simulink model "ROS2ValetVehicleExample"  (R2022b)
settings: Solver=FixedStepAuto  StartTime=0.0  StopTime=inf  FixedStep=0.05  MaxStep=1e-2  MinStep=1e-3  RelTol=5e-3
StopFcn:
  | exampleHelperROSValetModelCallbacks('stopfcn');
model workspace (MAT data in the model file):
  SL_ROS_VariableLengthArrays_MaxSizes.CommonInfo.ArrayTruncateAction = 'EmitWarning'
  SL_ROS_VariableLengthArrays_MaxSizes.MsgTypeMap = containers.Map
  SL_ROS_VariableLengthArrays_MaxSizes.MsgTypeMap.serialization.keys = {'std_msgs/Float64MultiArray'}
  SL_ROS_VariableLengthArrays_MaxSizes.MsgTypeMap.serialization.values{1}.PropertyName = 'data'
  SL_ROS_VariableLengthArrays_MaxSizes.MsgTypeMap.serialization.values{1}.DataType = 'double'
  SL_ROS_VariableLengthArrays_MaxSizes.MsgTypeMap.serialization.values{1}.MaxLength = 1500
  SL_ROS_VariableLengthArrays_MaxSizes.MsgTypeMap.serialization.uniformity = 0
  SL_ROS_VariableLengthArrays_MaxSizes.MsgTypeMap.serialization.keyType = 'char'
  SL_ROS_VariableLengthArrays_MaxSizes.MsgTypeMap.serialization.valueType = 'any'
values from neighbouring files (symbols this model uses):
  costmapStruct = rmfield(costmapStruct, 'CollisionChecker')    [exampleHelperROSValetSLCreateUtilityStruct.m]
  vehicleDimsStruct = exampleHelperROSValetMatchStructFields(vehicleDimsStruct, obj.CollisionChecker.VehicleDimensions)    [exampleHelperROSValetSLCreateUtilityStruct.m]
undefined symbols (not defined in the file or in its folder): startPose, theta, x, y
libraries: ros2lib x15, simulink x2, simulink_extras x2, helperVarsizeLib x1, autolibshared x1
CloseFcn:
  | exampleHelperROSValetModelCallbacks('closefcn');
settings Model: Creator=The MathWorks, Inc.  LastModifiedBy=The MathWorks, Inc.
settings SolverCC: ZeroCrossAlgorithm=Adaptive  AlgebraicLoopSolver=TrustRegion
settings OptimizationCC: EnhancedBackFolding=on  PassReuseOutputArgsThreshold=0  ZeroExternalMemoryAtStartup=off  ZeroInternalMemoryAtStartup=off  MaxStackSize=64  OptimizeBlockOrder=speed  DifferentSizesBufferReuse=on  OptimizationCustomize=off
settings DebuggingCC: ParameterTunabilityLossMsg=error  UnconnectedInputMsg=warning  UnconnectedOutputMsg=warning  UnconnectedLineMsg=warning  SFMachineParentedDataDiag=warning
settings HardwareCC: UseEmbeddedCoderFeatures=off
settings ModelReferenceCC: EnableRefExpFcnMdlSchedulingChecks=on
settings SFSimCC: MATLABDynamicMemAlloc=off  SimTargetLang=C++
settings RTWCC: Description=Embedded Coder  SystemTargetFile=ert.tlc  HardwareBoard=Robot Operating System 2 (ROS 2)  TLCOptions=-aInlineSetEventsForThisBaseRateFcn=TLC_FALSE -aSuppressMultiTaskScheduler=TLC_FALSE -aRateBasedStepFcn=1  TemplateMakefile=ert_default_tmf  GenerateReport=on  Toolchain=Colcon Tools  LaunchReport=on  TargetLang=C++
settings CodeAppCC: ForceParamTrailComments=on  OperatorAnnotations=on
settings ERTTargetCC: ERTCustomFileBanners=off  CodeInterfacePackaging=C++ class  SupportContinuousTime=on  SupportNonInlinedSFcns=on  RemoveResetFunc=off  ModelStepFunctionPrototypeControlCompliant=off  RootIOFormat=Structure reference

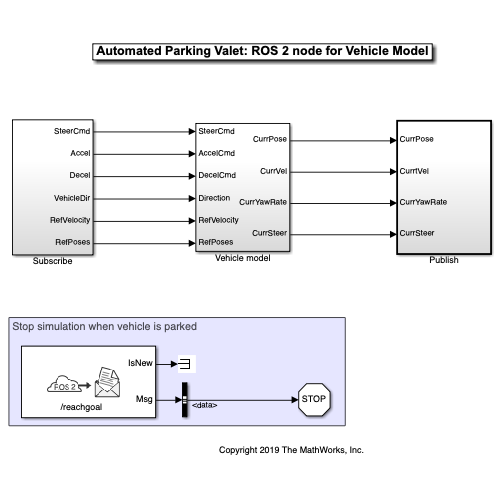
[thumbnail: Simulink's stored preview of the top-level diagram]
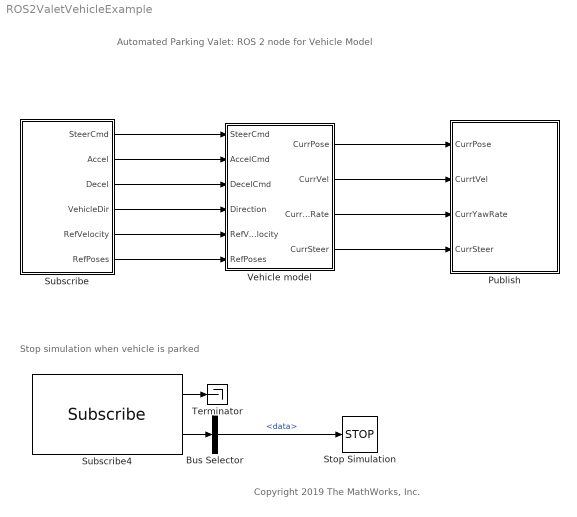
== system ROS2ValetVehicleExample ==
  note: Automated Parking Valet: ROS 2 node for Vehicle Model
  note: Copyright 2019 The MathWorks, Inc.
  note: Stop simulation when vehicle is parked
  Bus Selector : BusSelector  OutputSignals=data
  Publish : Subsystem  TreatAsAtomicUnit=on
  Stop Simulation : Stop
  Subscribe : Subsystem  SystemSampleTime=0.01
  Subscribe4 : ros2lib/Subscribe  topicSource=Specify your own  topic=/reachgoal  messageType=std_msgs/Bool  sampleTime=-1  QOSHistory=Keep last  QOSDepth=1  QOSReliability=Reliable  QOSDurability=Volatile
  Terminator : Terminator
  Vehicle model : Subsystem
  wires:
  Subscribe/1(SteerCmd) -> Vehicle model/1(SteerCmd)
  Subscribe/2(Accel) -> Vehicle model/2(AccelCmd)
  Subscribe/3(Decel) -> Vehicle model/3(DecelCmd)
  Subscribe/4(VehicleDir) -> Vehicle model/4(Direction)
  Subscribe/6(RefPoses) -> Vehicle model/6(RefPoses)
  Subscribe/5(RefVelocity) -> Vehicle model/5(RefVelocity)
  Vehicle model/1(CurrPose) -> Publish/1(CurrPose)
  Vehicle model/2(CurrVel) -> Publish/2(CurrtVel)
  Vehicle model/3(CurrYawRate) -> Publish/3(CurrYawRate)
  Vehicle model/4(CurrSteer) -> Publish/4(CurrSteer)
  Bus Selector/1 -> Stop Simulation/1  "<data>"
  Subscribe4/1 -> Terminator/1
  Subscribe4/2 -> Bus Selector/1

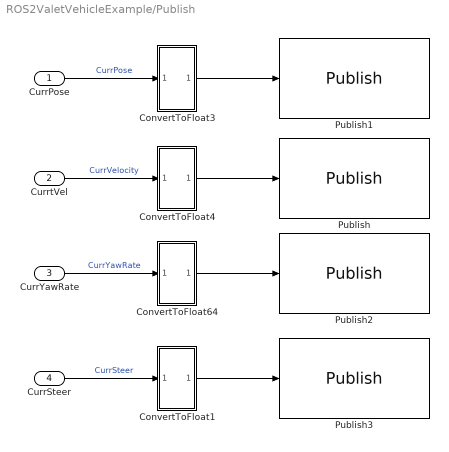
== system ROS2ValetVehicleExample/Publish ==
  CurrPose : Inport
  CurrtVel : Inport  Port=2
  CurrYawRate : Inport  Port=3
  CurrSteer : Inport  Port=4
  ConvertToFloat1 : Subsystem
  ConvertToFloat3 : Subsystem
  ConvertToFloat4 : Subsystem
  ConvertToFloat64 : Subsystem
  Publish : ros2lib/Publish  topicSource=Specify your own  topic=/currentvel  messageType=std_msgs/Float64  QOSHistory=Keep last  QOSDepth=1  QOSReliability=Reliable  QOSDurability=Volatile
  Publish1 : ros2lib/Publish  topicSource=Specify your own  topic=/currentpose  messageType=geometry_msgs/Pose2D  QOSHistory=Keep last  QOSDepth=1  QOSReliability=Reliable  QOSDurability=Volatile
  Publish2 : ros2lib/Publish  topicSource=Specify your own  topic=/curryawrate  messageType=std_msgs/Float64  QOSHistory=Keep last  QOSDepth=1  QOSReliability=Reliable  QOSDurability=Volatile
  Publish3 : ros2lib/Publish  topicSource=Specify your own  topic=/currentsteering  messageType=std_msgs/Float64  QOSHistory=Keep last  QOSDepth=1  QOSReliability=Reliable  QOSDurability=Volatile
  wires:
  ConvertToFloat4/1(Out1) -> Publish/1
  CurrYawRate/1 -> ConvertToFloat64/1(In1)  "CurrYawRate"
  ConvertToFloat64/1(Out1) -> Publish2/1
  ConvertToFloat1/1(Out1) -> Publish3/1
  CurrPose/1 -> ConvertToFloat3/1(In1)  "CurrPose"
  CurrSteer/1 -> ConvertToFloat1/1(In1)  "CurrSteer"
  ConvertToFloat3/1(Out1) -> Publish1/1
  CurrtVel/1 -> ConvertToFloat4/1(In1)  "CurrVelocity"

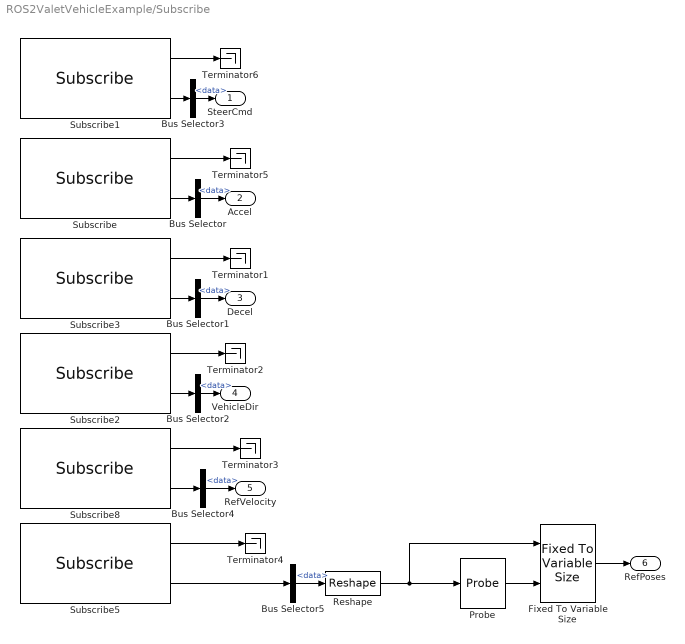
== system ROS2ValetVehicleExample/Subscribe ==
  Bus Selector{,1..5} (6 alike) : BusSelector  OutputSignals=data
  Fixed To Variable Size : helperVarsizeLib/Fixed To Variable Size  SystemSampleTime=-1  VariantActivationTime=update diagram  Latency=0  AutoFrameSizeCalculation=off
  Probe : Probe  ProbeWidth=off  ProbeSampleTime=off  ProbeComplexSignal=off  ProbeSignalDimensions=on
  Reshape : Reshape  OutputDimensionality=Customize  OutputDimensions=[500,3]
  Subscribe : ros2lib/Subscribe  topicSource=Specify your own  topic=/accelcmd  messageType=std_msgs/Float64  sampleTime=-1  QOSHistory=Keep last  QOSDepth=1  QOSReliability=Reliable  QOSDurability=Volatile
  Subscribe1 : ros2lib/Subscribe  topicSource=Specify your own  topic=/steeringangle  messageType=std_msgs/Float64  sampleTime=-1  QOSHistory=Keep last  QOSDepth=1  QOSReliability=Reliable  QOSDurability=Volatile
  Subscribe2 : ros2lib/Subscribe  topicSource=Select from ROS network  topic=/vehdir  messageType=std_msgs/Float64  sampleTime=-1  QOSHistory=Keep last  QOSDepth=1  QOSReliability=Reliable  QOSDurability=Volatile
  Subscribe3 : ros2lib/Subscribe  topicSource=Specify your own  topic=/decelcmd  messageType=std_msgs/Float64  sampleTime=-1  QOSHistory=Keep last  QOSDepth=1  QOSReliability=Reliable  QOSDurability=Volatile
  Subscribe5 : ros2lib/Subscribe  topicSource=Specify your own  topic=/smoothpath  messageType=std_msgs/Float64MultiArray  sampleTime=-1  QOSHistory=Keep last  QOSDepth=1  QOSReliability=Reliable  QOSDurability=Volatile
  Subscribe8 : ros2lib/Subscribe  topicSource=Specify your own  topic=/refvelocity  messageType=std_msgs/Float64  sampleTime=-1  QOSHistory=Keep last  QOSDepth=1  QOSReliability=Reliable  QOSDurability=Volatile
  Terminator{1..6} (6 alike) : Terminator
  SteerCmd : Outport  VectorParamsAs1DForOutWhenUnconnected=off
  Accel : Outport  Port=2  VectorParamsAs1DForOutWhenUnconnected=off
  Decel : Outport  Port=3  VectorParamsAs1DForOutWhenUnconnected=off
  VehicleDir : Outport  Port=4  VectorParamsAs1DForOutWhenUnconnected=off
  RefVelocity : Outport  Port=5  VectorParamsAs1DForOutWhenUnconnected=off
  RefPoses : Outport  Port=6  VectorParamsAs1DForOutWhenUnconnected=off
  wires:
  Subscribe/2 -> Bus Selector/1
  Subscribe3/2 -> Bus Selector1/1
  Subscribe2/2 -> Bus Selector2/1
  Subscribe1/2 -> Bus Selector3/1
  Subscribe5/2 -> Bus Selector5/1
  Subscribe8/2 -> Bus Selector4/1
  Bus Selector3/1 -> SteerCmd/1  "<data>"
  Bus Selector/1 -> Accel/1  "<data>"
  Bus Selector1/1 -> Decel/1  "<data>"
  Bus Selector2/1 -> VehicleDir/1  "<data>"
  Bus Selector4/1 -> RefVelocity/1  "<data>"
  Reshape/1 -> Fixed To Variable Size/1, Probe/1
  Probe/1 -> Fixed To Variable Size/2
  Bus Selector5/1 -> Reshape/1  "<data>"
  Fixed To Variable Size/1 -> RefPoses/1
  Subscribe2/1 -> Terminator2/1
  Subscribe8/1 -> Terminator3/1
  Subscribe5/1 -> Terminator4/1
  Subscribe3/1 -> Terminator1/1
  Subscribe/1 -> Terminator5/1
  Subscribe1/1 -> Terminator6/1

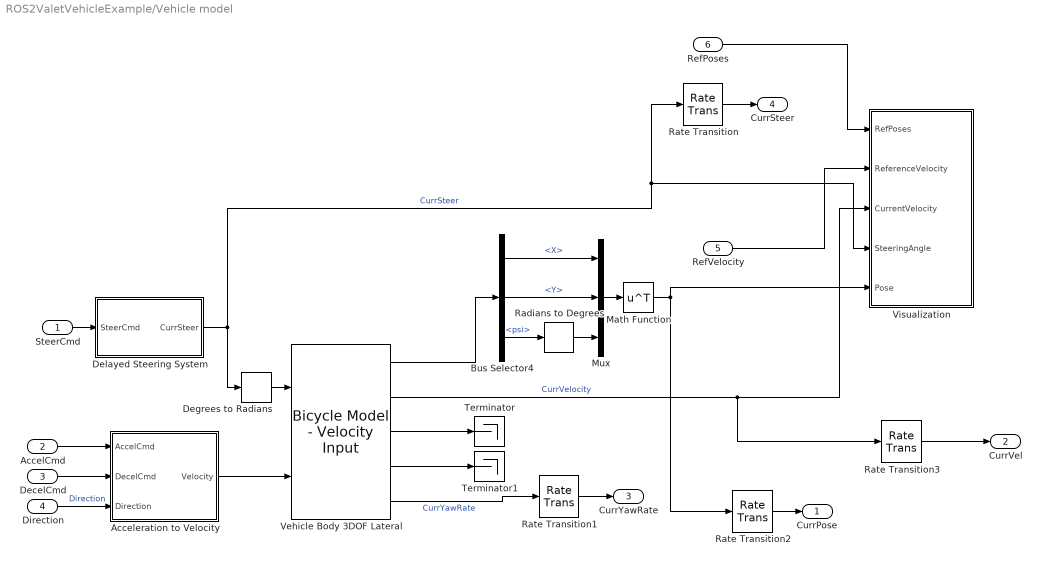
== system ROS2ValetVehicleExample/Vehicle model ==
  SteerCmd : Inport
  AccelCmd : Inport  Port=2
  DecelCmd : Inport  Port=3
  Direction : Inport  Port=4
  RefVelocity : Inport  Port=5
  RefPoses : Inport  Port=6
  Acceleration to Velocity : Subsystem  TreatAsAtomicUnit=on
  Bus Selector4 : BusSelector  OutputSignals=InertFrm.RearAxl.Disp.X,InertFrm.RearAxl.Disp.Y,InertFrm.Cg.Ang.psi
  Degrees to Radians : simulink_extras/Transformations/Degrees to Radians
  Delayed Steering System : Subsystem
  Math Function : Math  Operator=transpose  SignedPower=on
  Mux : Mux  Inputs=3
  Radians to Degrees : simulink_extras/Transformations/Radians to Degrees
  Rate Transition{,1..3} (4 alike) : RateTransition
  Terminator : Terminator
  Terminator1 : Terminator
  Vehicle Body 3DOF Lateral : autolibshared/Bicycle Model - Velocity Input  trackMode=Single (bicycle)  inputMode=External longitudinal forces  frontSteerMode=on  rearSteerMode=off  windMode=off  muMode=off  extFMode=off  extMMode=off  aMode=3  NF=2  NR=2  m=1575  a=1.2  b=1.6  h=0.35  X_o=startPose(1)+cosd(startPose(3))*1.6  xdot_o=0  CalphaMode=off  sigmaMode=on  w=[1.4,1.4]  Cy_f=19e3  Cy_r=20e3  sigma_f=.1  sigma_r=.1  alpha_f_brk=[-.1 .1]  Cy_f_data=[-9e3 9e3]  alpha_r_brk=[-.1 .1]  Cy_r_data=[-9e3 9e3]  Y_o=startPose(2) +sind(startPose(3))*1.6  ydot_o=0  Izz=4000  psi_o=deg2rad(startPose(3))  r_o=0  Af=2  Cd=.3  Cl=.1  Cpm=.1  beta_w=[0:0.01:0.3]  Cs=[0:0.03:0.9]  Cym=[0:0.01:0.3]  Pabs=101325  Tair=273  g=9.81  mu=1  xdot_tol=0.01  Fznom=5000  Fxtire_sat=1e6  Fytire_sat=1e6  longOff=0  latOff=0  vertOff=0
  Visualization : Subsystem
  CurrPose : Outport
  CurrVel : Outport  Port=2
  CurrYawRate : Outport  Port=3
  CurrSteer : Outport  Port=4
  wires:
  Degrees to Radians/1 -> Vehicle Body 3DOF Lateral/1
  Delayed Steering System/1(CurrSteer) -> Rate Transition/1, Visualization/4(SteeringAngle), Degrees to Radians/1  "CurrSteer"
  Acceleration to Velocity/1(Velocity) -> Vehicle Body 3DOF Lateral/2
  AccelCmd/1 -> Acceleration to Velocity/1(AccelCmd)
  DecelCmd/1 -> Acceleration to Velocity/2(DecelCmd)
  SteerCmd/1 -> Delayed Steering System/1(SteerCmd)
  RefPoses/1 -> Visualization/1(RefPoses)
  RefVelocity/1 -> Visualization/2(ReferenceVelocity)
  Bus Selector4/3 -> Radians to Degrees/1  "<psi>"
  Vehicle Body 3DOF Lateral/3 -> Terminator/1
  Bus Selector4/1 -> Mux/1  "<X>"
  Bus Selector4/2 -> Mux/2  "<Y>"
  Radians to Degrees/1 -> Mux/3
  Mux/1 -> Math Function/1
  Vehicle Body 3DOF Lateral/4 -> Terminator1/1
  Direction/1 -> Acceleration to Velocity/3(Direction)  "Direction"
  Vehicle Body 3DOF Lateral/5 -> Rate Transition1/1  "CurrYawRate"
  Vehicle Body 3DOF Lateral/2 -> Rate Transition3/1, Visualization/3(CurrentVelocity)  "CurrVelocity"
  Vehicle Body 3DOF Lateral/1 -> Bus Selector4/1
  Math Function/1 -> Rate Transition2/1, Visualization/5(Pose)
  Rate Transition/1 -> CurrSteer/1
  Rate Transition1/1 -> CurrYawRate/1
  Rate Transition2/1 -> CurrPose/1
  Rate Transition3/1 -> CurrVel/1

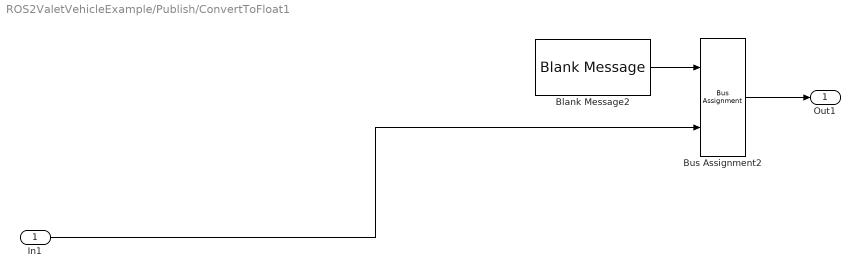
== system ROS2ValetVehicleExample/Publish/ConvertToFloat1 ==
  In1 : Inport
  Blank Message2 : ros2lib/Blank Message  messageClass=Message  entityType=std_msgs/Float64  messageType=std_msgs/Float64  SampleTime=inf
  Bus Assignment2 : BusAssignment  AssignedSignals=data
  Out1 : Outport
  wires:
  In1/1 -> Bus Assignment2/2
  Bus Assignment2/1 -> Out1/1
  Blank Message2/1 -> Bus Assignment2/1

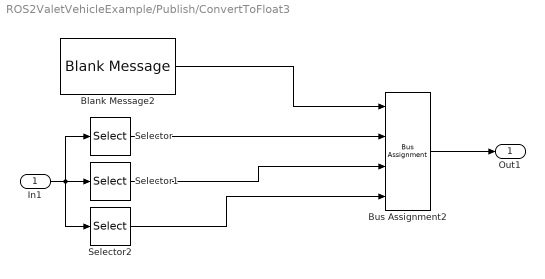
== system ROS2ValetVehicleExample/Publish/ConvertToFloat3 ==
  In1 : Inport
  Blank Message2 : ros2lib/Blank Message  messageClass=Message  entityType=geometry_msgs/Pose2D  messageType=geometry_msgs/Pose2D  SampleTime=inf
  Bus Assignment2 : BusAssignment  AssignedSignals=x,y,theta
  Selector : Selector  InputPortWidth=3  IndexOptions=Index vector (dialog)  Indices=1  OutputSizes=1
  Selector1 : Selector  InputPortWidth=3  IndexOptions=Index vector (dialog)  Indices=2  OutputSizes=1
  Selector2 : Selector  InputPortWidth=3  IndexOptions=Index vector (dialog)  Indices=3  OutputSizes=1
  Out1 : Outport
  wires:
  Bus Assignment2/1 -> Out1/1
  Blank Message2/1 -> Bus Assignment2/1
  In1/1 -> Selector2/1, Selector1/1, Selector/1
  Selector/1 -> Bus Assignment2/2
  Selector1/1 -> Bus Assignment2/3
  Selector2/1 -> Bus Assignment2/4

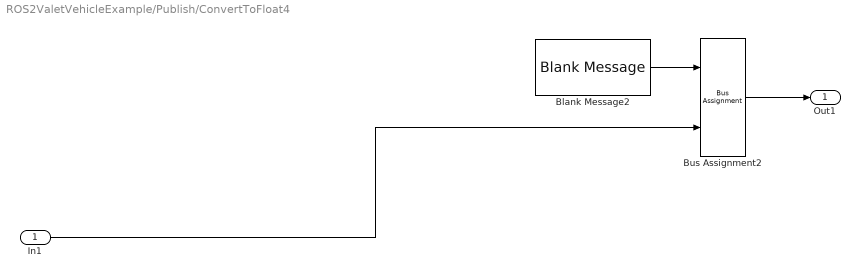
== system ROS2ValetVehicleExample/Publish/ConvertToFloat4 ==
  In1 : Inport
  Blank Message2 : ros2lib/Blank Message  messageClass=Message  entityType=std_msgs/Float64  messageType=std_msgs/Float64  SampleTime=inf
  Bus Assignment2 : BusAssignment  AssignedSignals=data
  Out1 : Outport
  wires:
  In1/1 -> Bus Assignment2/2
  Bus Assignment2/1 -> Out1/1
  Blank Message2/1 -> Bus Assignment2/1

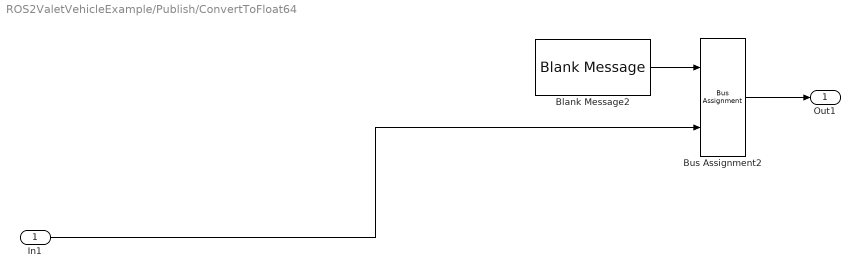
== system ROS2ValetVehicleExample/Publish/ConvertToFloat64 ==
  In1 : Inport
  Blank Message2 : ros2lib/Blank Message  messageClass=Message  entityType=std_msgs/Float64  messageType=std_msgs/Float64  SampleTime=inf
  Bus Assignment2 : BusAssignment  AssignedSignals=data
  Out1 : Outport
  wires:
  Blank Message2/1 -> Bus Assignment2/1
  Bus Assignment2/1 -> Out1/1
  In1/1 -> Bus Assignment2/2

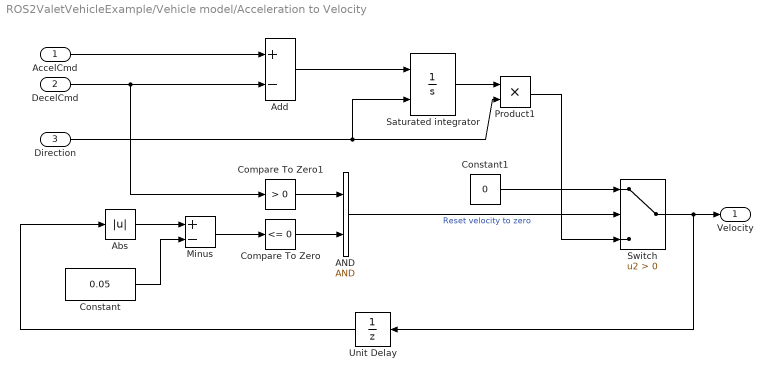
== system ROS2ValetVehicleExample/Vehicle model/Acceleration to Velocity ==
  AccelCmd : Inport  PortDimensions=[1 1]
  DecelCmd : Inport  Port=2  PortDimensions=[1 1]
  Direction : Inport  Port=3
  AND : Logic  IconShape=distinctive  AllPortsSameDT=off  OutDataTypeStr=boolean
  Abs : Abs  SaturateOnIntegerOverflow=off
  Add : Sum  Inputs=+-
  Compare To Zero : simulink/Logic and Bit Operations/Compare To Zero  relop=<=  OutDataTypeStr=boolean
  Compare To Zero1 : simulink/Logic and Bit Operations/Compare To Zero  relop=>  OutDataTypeStr=boolean
  Constant : Constant  Value=0.05
  Constant1 : Constant  Value=0
  Minus : Sum  Inputs=+-
  Product1 : Product
  Saturated integrator : Integrator  ExternalReset=either  LimitOutput=on  LowerSaturationLimit=0  AbsoluteTolerance=1e-3  ZeroCross=off
  Switch : Switch  Criteria=u2 > Threshold  SaturateOnIntegerOverflow=off  InputSameDT=off
  Unit Delay : UnitDelay  SampleTime=-1  HasFrameUpgradeWarning=on
  Velocity : Outport  VectorParamsAs1DForOutWhenUnconnected=off
  wires:
  Direction/1 -> Product1/2, Saturated integrator/2
  AccelCmd/1 -> Add/1
  Add/1 -> Saturated integrator/1
  DecelCmd/1 -> Compare To Zero1/1, Add/2
  Unit Delay/1 -> Abs/1
  Abs/1 -> Minus/1
  Constant/1 -> Minus/2
  Minus/1 -> Compare To Zero/1
  Compare To Zero/1 -> AND/2
  Compare To Zero1/1 -> AND/1
  AND/1 -> Switch/2  "Reset velocity to zero"
  Switch/1 -> Unit Delay/1, Velocity/1
  Constant1/1 -> Switch/1
  Saturated integrator/1 -> Product1/1
  Product1/1 -> Switch/3

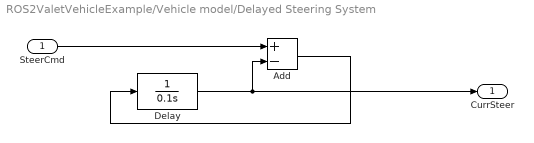
== system ROS2ValetVehicleExample/Vehicle model/Delayed Steering System ==
  SteerCmd : Inport
  Add : Sum  Inputs=+-
  Delay : TransferFcn  Denominator=[0.1 0]
  CurrSteer : Outport  VectorParamsAs1DForOutWhenUnconnected=off
  wires:
  Add/1 -> Delay/1
  SteerCmd/1 -> Add/1
  Delay/1 -> CurrSteer/1, Add/2

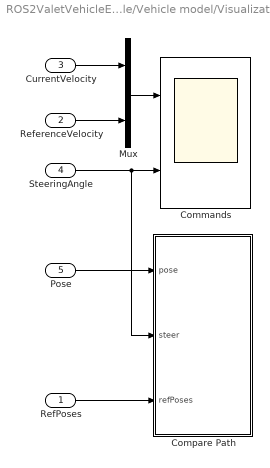
== system ROS2ValetVehicleExample/Vehicle model/Visualization ==
  RefPoses : Inport
  ReferenceVelocity : Inport  Port=2
  CurrentVelocity : Inport  Port=3
  SteeringAngle : Inport  Port=4
  Pose : Inport  Port=5
  Commands : Scope  NumInputPorts=2
  Compare Path : MATLAB Function  TreatAsAtomicUnit=on
  Mux : Mux  Inputs=2
  wires:
  CurrentVelocity/1 -> Mux/1
  SteeringAngle/1 -> Compare Path/2(steer), Commands/2
  RefPoses/1 -> Compare Path/3(refPoses)
  Mux/1 -> Commands/1
  ReferenceVelocity/1 -> Mux/2
  Pose/1 -> Compare Path/1(pose)

== matlab function ROS2ValetVehicleExample/Vehicle model/Visualization/Compare Path ==
  settings: updateMethod=DISCRETE  sampleTime=0.1
  data: pose input size=[1 3]; steer input; refPoses input; costmapStruct parameter; vehicleDimsStruct parameter
function visualizePath(pose, steer, refPoses, costmapStruct, vehicleDimsStruct)

%visualizePath Display simulation results.

coder.extrinsic('exampleHelperROSValetSLVisualizePath');

exampleHelperROSValetSLVisualizePath(pose, steer, refPoses, costmapStruct, vehicleDimsStruct)
